simulink model "FTC"  (R2025a)
settings: Solver=ode45  StartTime=0.0  StopTime=10  RelTol=1e-3  EnableMultiTasking=on
values from neighbouring files (symbols this model uses):
  A = [-0.64 1.51 -22.95 9.78 0 ... (first row only)    [thesis_final.m]
  B = [-1.25 3.19 ... (first row only)    [thesis_final.m]
  C = [0.04 0 0 0 0 ... (first row only)    [thesis_final.m]
  E = amp*ones(5,2)    [thesis_final.m]
  fault_type = input('1=abrupt fault ,2= incipient fault,3=intermittent fault:')    [thesis_final.m]
  L = (w*inv(l))'    [thesis_final.m]
  t_fault = input('simulation start time=0s, end time=10s:')    [thesis_final.m]
  W = W'    [thesis_final.m]
undefined symbols (not defined in the file or in its folder): Continuous, K, Kab, Kinc, Kint, Time
libraries: dspsrcs4 x14, simulink x5, ctrlSharedLib x4
settings Model: SimulationMode=accelerator  Creator=Qandeel Fazal  LastModifiedBy=VICTUS
settings SolverCC: MaxConsecutiveZCs=100000  ZeroCrossControl=DisableAll  ZeroCrossAlgorithm=Adaptive  AlgebraicLoopSolver=TrustRegion
settings DataIOCC: LimitDataPoints=on  SaveFormat=Array  ReturnWorkspaceOutputs=off
settings OptimizationCC: EfficientMapNaN2IntZero=off  LifeSpan=inf  SimCompilerOptimization=on
settings DebuggingCC: UnconnectedInputMsg=warning  UnconnectedOutputMsg=warning  UnconnectedLineMsg=warning  SFUnexpectedBacktrackingDiag=warning  SFNoUnconditionalDefaultTransitionDiag=warning  SFExecutionAtInitializationDiag=none  ArithmeticOperatorsInVariantConditions=warning
settings HardwareCC: ProdBitPerPointer=32.0  ProdBitPerSizeT=32.0  ProdBitPerPtrDiffT=32.0  ProdLargestAtomicFloat=None  ProdIntDivRoundTo=Undefined  ProdEndianess=Unspecified  ProdWordSize=32.0  ProdHWDeviceType=32-bit Generic  TargetBitPerPointer=64.0  TargetBitPerSizeT=64.0  TargetBitPerPtrDiffT=64.0  TargetLongLongMode=on  TargetIntDivRoundTo=Zero  TargetEndianess=LittleEndian  TargetWordSize=64.0  TargetHWDeviceType=MATLAB Host  ProdEqTarget=off
settings ModelReferenceCC: EnableRefExpFcnMdlSchedulingChecks=on  PropagateSignalLabelsOutOfModel=off
settings SFSimCC: SimUseLocalCustomCode=off  CustomCodeUndefinedFunction=UseInterfaceOnly
settings RTWCC: RTWUseLocalCustomCode=off  GPUComputeCapability=3.5
settings CodeAppCC: MaxIdLength=128.0  StateflowObjectComments=on
settings GRTTargetCC: TargetLangStandard=C89/C90 (ANSI)  CombineOutputUpdateFcns=off  GRTInterface=on
settings ConfigComp: CovMetricSettings=dw  CovSaveCumulativeToWorkspaceVar=on  CovSaveSingleToWorkspaceVar=on  CovExternalEMLEnable=off  CovSFcnEnable=off

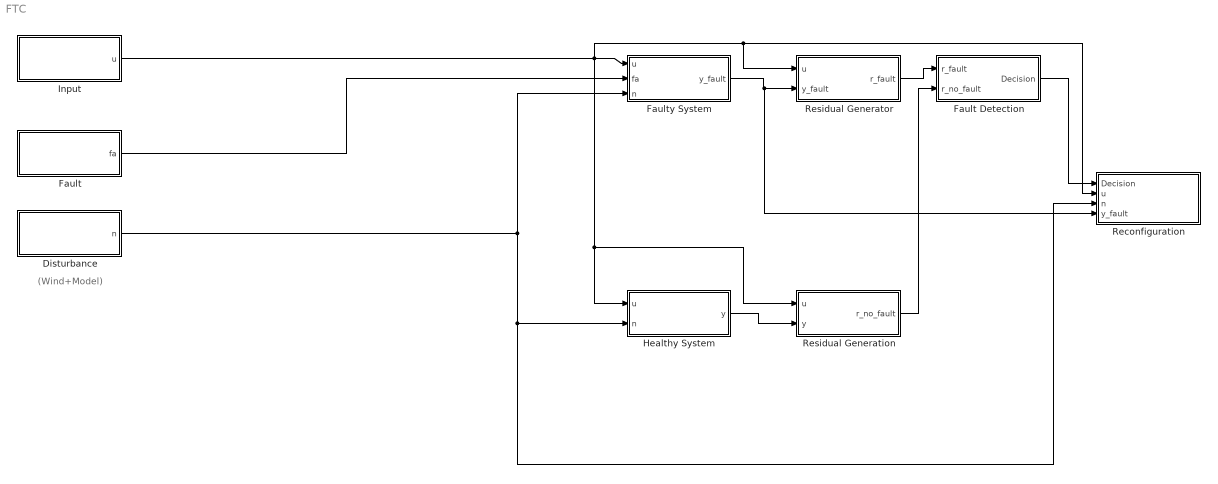
== system FTC ==
  note: (Wind+Model)
  Disturbance : Subsystem
  Fault : Subsystem
  Fault Detection : Subsystem
  Faulty System : Subsystem
  Healthy System : Subsystem
  Input : Subsystem
  Reconfiguration : Subsystem
  Residual Generation : Subsystem
  Residual Generator : Subsystem
  wires:
  Faulty System/1(y_fault) -> Reconfiguration/4(y_fault), Residual Generator/2(y_fault)
  Healthy System/1(y) -> Residual Generation/2(y)
  Fault/1(fa) -> Faulty System/2(fa)
  Residual Generator/1(r_fault) -> Fault Detection/1(r_fault)
  Residual Generation/1(r_no_fault) -> Fault Detection/2(r_no_fault)
  Fault Detection/1(Decision) -> Reconfiguration/1(Decision)
  Input/1(u) -> Reconfiguration/2(u), Residual Generator/1(u), Healthy System/1(u), Residual Generation/1(u), Faulty System/1(u)
  Disturbance/1(n) -> Healthy System/2(n), Reconfiguration/3(n), Faulty System/3(n)

== system FTC/Disturbance ==
  Mux : Mux  Inputs=2
  Scope2 : Scope  Commented=on
      settings: DataLoggingVariableName=ScopeData3  DataLoggingSaveFormat=Array
  To Workspace6 : ToWorkspace  VariableName=n  SaveFormat=Timeseries  SampleTime=-1
      settings: Save2DSignal=2-D array (concatenate along first dimension)
  n(1) : dspsrcs4/Random Source  SrcType=Gaussian  NormMethod=Ziggurat  CltLength=12  MinVal=0  MaxVal=1  MeanVal=0  VarVal=0.1  RepMode=Not repeatable  rawSeed=1  IsInherit=off  SampMode=Continuous  SampTime=1  SampFrame=1  DataType=Double  OutComplex=Real  OutputFrames=on
  n(2) : dspsrcs4/Random Source  SrcType=Gaussian  NormMethod=Ziggurat  CltLength=12  MinVal=0  MaxVal=1  MeanVal=0  VarVal=0.1  RepMode=Not repeatable  rawSeed=1  IsInherit=off  SampMode=Continuous  SampTime=1  SampFrame=1  DataType=Double  OutComplex=Real  OutputFrames=on
  n : Outport
  wires:
  Mux/1 -> n/1, To Workspace6/1, Scope2/1
  n(1)/1 -> Mux/1
  n(2)/1 -> Mux/2

== system FTC/Fault ==
  Constant : Constant  Value=fault_type
  Constant1 : Constant  Value=0
  Constant2 : Constant  Value=0
  Incipient Fault : simulink/Sources/Ramp  slope=1  start=t_fault  X0=0
  Intermittent Fault : DiscretePulseGenerator  PulseType=Time based  Period=3  PulseWidth=4  PhaseDelay=t_fault
  Multiport Switch : MultiPortSwitch  DataPortOrder=Specify indices  SaturateOnIntegerOverflow=off  InputSameDT=off
  Mux : Mux  Inputs=2
  Mux1 : Mux  Inputs=2
  Mux2 : Mux  Inputs=2
  Scope2 : Scope  Commented=on
      settings: DataLoggingVariableName=ScopeData3  DataLoggingSaveFormat=Array
  To Workspace6 : ToWorkspace  VariableName=fa  SaveFormat=Timeseries  SampleTime=-1
      settings: Save2DSignal=2-D array (concatenate along first dimension)
  fa(1) : Step  Time=t_fault  After=0.3  SampleTime=0  VectorParams1D=off
  fa(2) : Step  Time=t_fault  After=0.3  SampleTime=0
  fa : Outport
  wires:
  Mux/1 -> Multiport Switch/2
  fa(1)/1 -> Mux/1
  fa(2)/1 -> Mux/2
  Incipient Fault/1 -> Mux1/1
  Constant1/1 -> Mux1/2
  Multiport Switch/1 -> fa/1, Scope2/1, To Workspace6/1
  Intermittent Fault/1 -> Mux2/1
  Constant2/1 -> Mux2/2
  Mux2/1 -> Multiport Switch/4
  Mux1/1 -> Multiport Switch/3
  Constant/1 -> Multiport Switch/1

== system FTC/Fault Detection ==
  r_fault : Inport
  r_no_fault : Inport  Port=2
  MATLAB Function : MATLAB Function  TreatAsAtomicUnit=on
  Scope8 : Scope  Commented=on  NumInputPorts=4
      settings: TimeSpan=50  ActiveDisplayYMinimum=0  ActiveDisplayYMaximum=1  DataLoggingVariableName=ScopeData11  DataLoggingSaveFormat=Array
  To Workspace1 : ToWorkspace  VariableName=d3  SaveFormat=Timeseries  SampleTime=-1
      settings: Save2DSignal=2-D array (concatenate along first dimension)
  To Workspace2 : ToWorkspace  VariableName=d4  SaveFormat=Timeseries  SampleTime=-1
      settings: Save2DSignal=2-D array (concatenate along first dimension)
  To Workspace3 : ToWorkspace  VariableName=decision  SaveFormat=Timeseries  SampleTime=-1
      settings: Save2DSignal=2-D array (concatenate along first dimension)
  To Workspace5 : ToWorkspace  VariableName=d1  SaveFormat=Timeseries  SampleTime=-1
      settings: Save2DSignal=2-D array (concatenate along first dimension)
  To Workspace8 : ToWorkspace  VariableName=d2  SaveFormat=Timeseries  SampleTime=-1
      settings: Save2DSignal=2-D array (concatenate along first dimension)
  Decision : Outport
  wires:
  MATLAB Function/1(d1) -> Decision/1, To Workspace3/1, Scope8/1, To Workspace5/1
  MATLAB Function/2(d2) -> To Workspace8/1, Scope8/2
  MATLAB Function/3(d3) -> Scope8/3, To Workspace1/1
  MATLAB Function/4(d4) -> Scope8/4, To Workspace2/1
  r_fault/1 -> MATLAB Function/1(r_fault)
  r_no_fault/1 -> MATLAB Function/2(r_no_fault)

== system FTC/Faulty System ==
  u : Inport
  fa : Inport  Port=2
  n : Inport  Port=3
  Mux : Mux  Inputs=2
  Scope2 : Scope  Commented=on
      settings: DataLoggingSaveFormat=Array
  State-Space : StateSpace  A=A  B=[B E]  C=C  D=zeros(5,4)  InitialCondition=[0 ;0;0;0;0]
  Sum5 : Sum  Inputs=|++
  To Workspace6 : ToWorkspace  VariableName=y_fault  SaveFormat=Timeseries  SampleTime=-1
      settings: Save2DSignal=2-D array (concatenate along first dimension)
  y_fault : Outport
  wires:
  fa/1 -> Sum5/2
  Mux/1 -> State-Space/1
  u/1 -> Sum5/1
  Sum5/1 -> Mux/1
  State-Space/1 -> To Workspace6/1, Scope2/1, y_fault/1
  n/1 -> Mux/2

== system FTC/Healthy System ==
  u : Inport
  n : Inport  Port=2
  Mux1 : Mux  Inputs=2
  Scope4 : Scope  Commented=on
      settings: DataLoggingVariableName=ScopeData10  DataLoggingSaveFormat=Array
  State-Space1 : StateSpace  A=A  B=[B E]  C=C  D=zeros(5,4)  InitialCondition=[0 ;0;0;0;0]
  To Workspace4 : ToWorkspace  VariableName=y  SaveFormat=Timeseries  SampleTime=-1
      settings: Save2DSignal=2-D array (concatenate along first dimension)
  y : Outport
  wires:
  u/1 -> Mux1/1
  Mux1/1 -> State-Space1/1
  n/1 -> Mux1/2
  State-Space1/1 -> y/1, To Workspace4/1, Scope4/1

== system FTC/Input ==
  Scope2 : Scope  Commented=on
      settings: DataLoggingVariableName=ScopeData3  DataLoggingSaveFormat=Array
  To Workspace6 : ToWorkspace  VariableName=u  SaveFormat=Timeseries  SampleTime=-1
      settings: Save2DSignal=2-D array (concatenate along first dimension)
  u(1)1 : Step  Before=[0 0]  After=[5 5]  SampleTime=0
  u : Outport
  wires:
  u(1)1/1 -> Scope2/1, u/1, To Workspace6/1

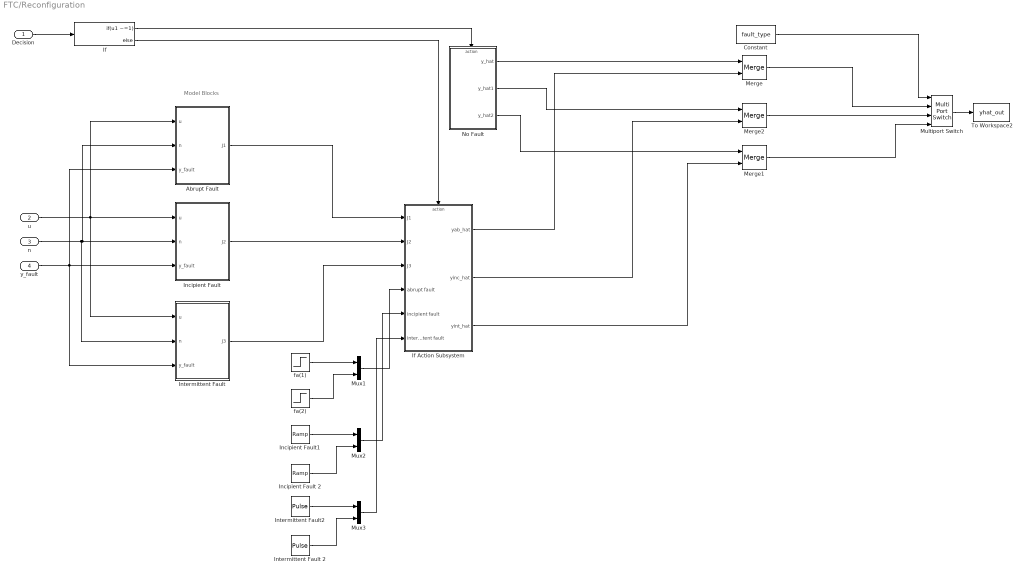
== system FTC/Reconfiguration ==
  note: Model Blocks
  Decision : Inport
  u : Inport  Port=2
  n : Inport  Port=3
  y_fault : Inport  Port=4
  Abrupt Fault : Subsystem
  Constant : Constant  Value=fault_type
  If : If  IfExpression=u1 ~=1
  If Action Subsystem : Subsystem  TreatAsAtomicUnit=on
  Incipient Fault : Subsystem
  Incipient Fault 2 : simulink/Sources/Ramp  slope=0  start=t_fault  InitialOutput=0
  Incipient Fault1 : simulink/Sources/Ramp  slope=1  start=5  InitialOutput=0
  Intermittent Fault : Subsystem
  Intermittent Fault 2 : DiscretePulseGenerator  PulseType=Time based  Amplitude=0  Period=10  PulseWidth=5
  Intermittent Fault2 : DiscretePulseGenerator  PulseType=Time based  PulseWidth=1.5  PhaseDelay=5
  Merge : Merge
  Merge1 : Merge
  Merge2 : Merge
  Multiport Switch : MultiPortSwitch  DataPortOrder=Specify indices  SaturateOnIntegerOverflow=off  InputSameDT=off
  Mux1 : Mux  Inputs=2
  Mux2 : Mux  Inputs=2
  Mux3 : Mux  Inputs=2
  No Fault : Subsystem  TreatAsAtomicUnit=on
  To Workspace2 : ToWorkspace  VariableName=yhat_out  SaveFormat=Timeseries  SampleTime=-1
  fa(1) : Step  Time=5  After=0.3  SampleTime=0  VectorParams1D=off
  fa(2) : Step  Time=t_fault  After=0  SampleTime=0
  wires:
  Decision/1 -> If/1
  If/2 -> If Action Subsystem/Action
  If/1 -> No Fault/Action
  Intermittent Fault/1(J3) -> If Action Subsystem/3(J3)
  u/1 -> Intermittent Fault/1(u), Abrupt Fault/1(u), Incipient Fault/1(u)
  n/1 -> Intermittent Fault/2(n), Abrupt Fault/2(n), Incipient Fault/2(n)
  y_fault/1 -> Intermittent Fault/3(y_fault), Abrupt Fault/3(y_fault), Incipient Fault/3(y_fault)
  Incipient Fault/1(J2) -> If Action Subsystem/2(J2)
  Abrupt Fault/1(J1) -> If Action Subsystem/1(J1)
  If Action Subsystem/1(yab_hat) -> Merge/2
  No Fault/1(y_hat) -> Merge/1
  If Action Subsystem/2(yinc_hat) -> Merge2/2
  No Fault/2(y_hat1) -> Merge2/1
  If Action Subsystem/3(yint_hat) -> Merge1/2
  No Fault/3(y_hat2) -> Merge1/1
  Constant/1 -> Multiport Switch/1
  Merge/1 -> Multiport Switch/2
  Merge2/1 -> Multiport Switch/3
  Merge1/1 -> Multiport Switch/4
  Multiport Switch/1 -> To Workspace2/1
  Mux1/1 -> If Action Subsystem/4(abrupt fault)
  fa(1)/1 -> Mux1/1
  fa(2)/1 -> Mux1/2
  Incipient Fault1/1 -> Mux2/1
  Incipient Fault 2/1 -> Mux2/2
  Intermittent Fault2/1 -> Mux3/1
  Intermittent Fault 2/1 -> Mux3/2
  Mux3/1 -> If Action Subsystem/6(intermittent fault)
  Mux2/1 -> If Action Subsystem/5(incipient fault)

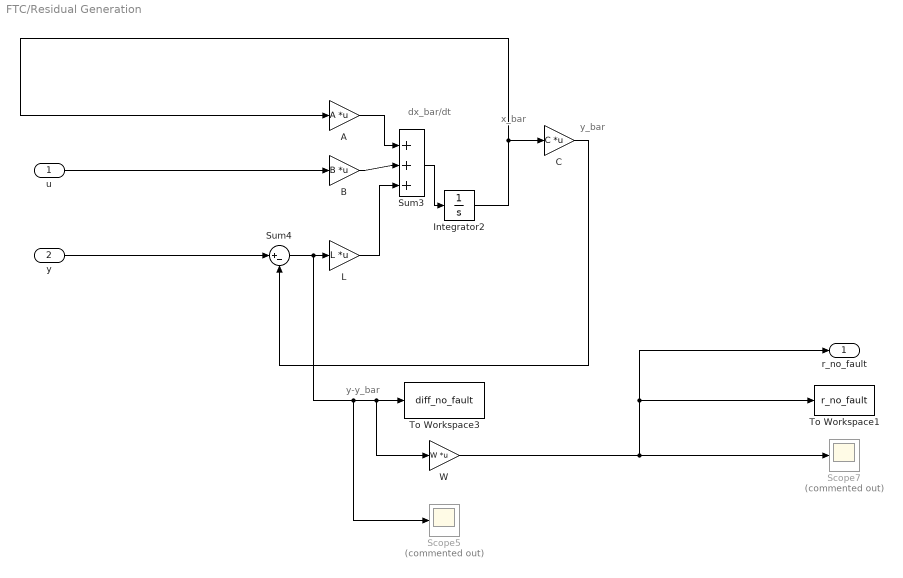
== system FTC/Residual Generation ==
  note: y-y_bar
  note: y_bar
  note: x_bar
  note: dx_bar/dt
  u : Inport
  y : Inport  Port=2
  "A " : Gain  Gain=A  Multiplication=Matrix(K*u)
  B : Gain  Gain=B  Multiplication=Matrix(K*u)
  C : Gain  Gain=C  Multiplication=Matrix(K*u)
  Integrator2 : Integrator
  "L " : Gain  Gain=L  Multiplication=Matrix(K*u)
  Scope5 : Scope  Commented=on
      settings: TimeSpan=50  ActiveDisplayYMinimum=-0.4  ActiveDisplayYMaximum=0.4  DataLoggingVariableName=ScopeData12  DataLoggingSaveFormat=Array
  Scope7 : Scope  Commented=on
      settings: TimeSpan=50  ActiveDisplayYMinimum=-0.4  ActiveDisplayYMaximum=0.80000000000000016  DataLoggingVariableName=ScopeData13  DataLoggingSaveFormat=Array
  Sum3 : Sum  Inputs=|+++
  Sum4 : Sum  Inputs=|+-
  To Workspace1 : ToWorkspace  VariableName=r_no_fault  SaveFormat=Timeseries  SampleTime=-1
      settings: Save2DSignal=2-D array (concatenate along first dimension)
  To Workspace3 : ToWorkspace  VariableName=diff_no_fault  SaveFormat=Timeseries  SampleTime=-1
      settings: Save2DSignal=2-D array (concatenate along first dimension)
  W : Gain  Gain=W  Multiplication=Matrix(K*u)
  r_no_fault : Outport
  wires:
  u/1 -> B/1
  B/1 -> Sum3/2
  "A "/1 -> Sum3/1
  C/1 -> Sum4/2
  Sum3/1 -> Integrator2/1
  "L "/1 -> Sum3/3
  Integrator2/1 -> C/1, "A "/1
  y/1 -> Sum4/1
  Sum4/1 -> Scope5/1, W/1, To Workspace3/1, "L "/1
  W/1 -> Scope7/1, r_no_fault/1, To Workspace1/1

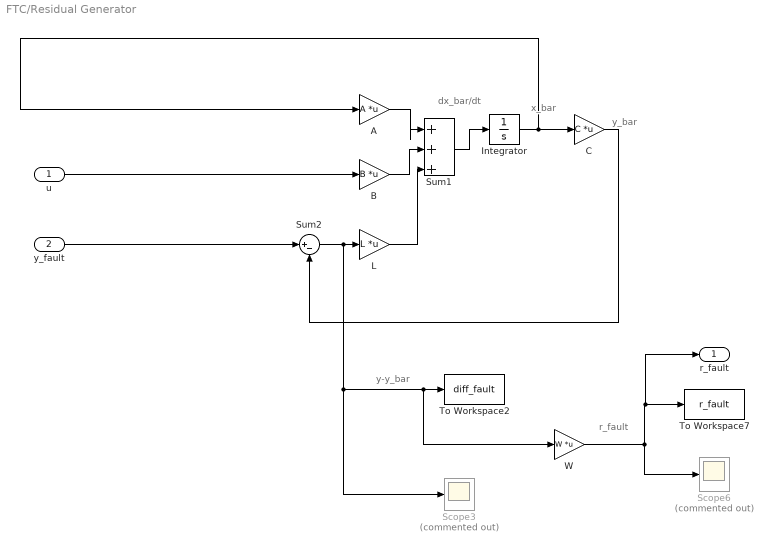
== system FTC/Residual Generator ==
  note: y_bar
  note: y-y_bar
  note: x_bar
  note: dx_bar/dt
  note: r_fault
  u : Inport
  y_fault : Inport  Port=2
  A : Gain  Gain=A  Multiplication=Matrix(K*u)
  B : Gain  Gain=B  Multiplication=Matrix(K*u)
  C : Gain  Gain=C  Multiplication=Matrix(K*u)
  Integrator : Integrator
  L : Gain  Gain=L  Multiplication=Matrix(K*u)
  Scope3 : Scope  Commented=on
      settings: TimeSpan=50  ActiveDisplayYMinimum=-0.4  ActiveDisplayYMaximum=0.80000000000000016  DataLoggingSaveFormat=Array
  Scope6 : Scope  Commented=on
      settings: TimeSpan=50  ActiveDisplayYMinimum=-100  ActiveDisplayYMaximum=600  DataLoggingVariableName=ScopeData9  DataLoggingSaveFormat=Array
  Sum1 : Sum  Inputs=|+++
  Sum2 : Sum  Inputs=|+-
  To Workspace2 : ToWorkspace  VariableName=diff_fault  SaveFormat=Timeseries  SampleTime=-1
      settings: Save2DSignal=2-D array (concatenate along first dimension)
  To Workspace7 : ToWorkspace  VariableName=r_fault  SaveFormat=Timeseries  SampleTime=-1
      settings: Save2DSignal=2-D array (concatenate along first dimension)
  W : Gain  Gain=W  Multiplication=Matrix(K*u)
  r_fault : Outport
  wires:
  B/1 -> Sum1/2
  A/1 -> Sum1/1
  C/1 -> Sum2/2
  Sum1/1 -> Integrator/1
  L/1 -> Sum1/3
  Integrator/1 -> C/1, A/1
  Sum2/1 -> W/1, To Workspace2/1, Scope3/1, L/1
  y_fault/1 -> Sum2/1
  u/1 -> B/1
  W/1 -> Scope6/1, r_fault/1, To Workspace7/1

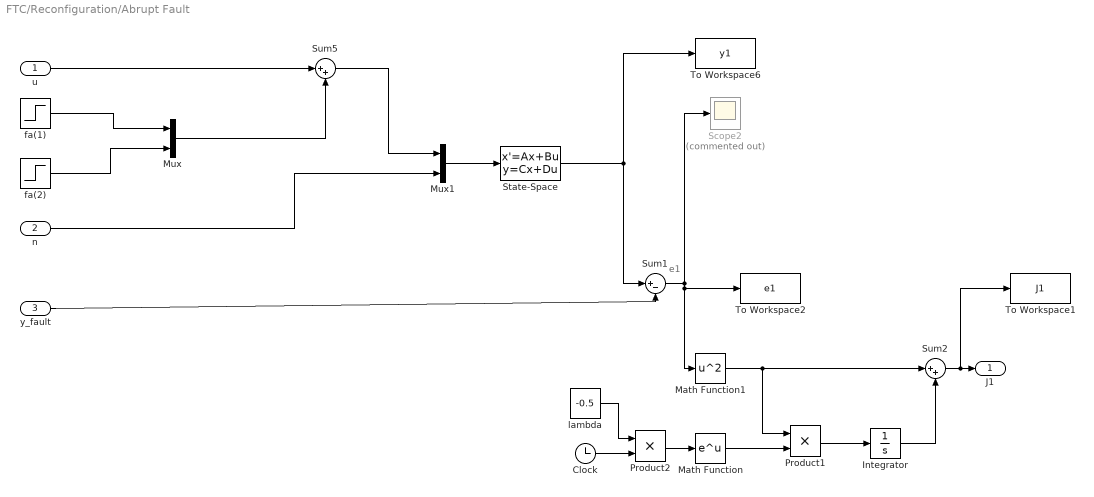
== system FTC/Reconfiguration/Abrupt Fault ==
  note: e1
  u : Inport
  n : Inport  Port=2
  y_fault : Inport  Port=3
  Clock : Clock
  Integrator : Integrator
  Math Function : Math  SignedPower=on
  Math Function1 : Math  Operator=square  SignedPower=on
  Mux : Mux  Inputs=2
  Mux1 : Mux  Inputs=2
  Product1 : Product
  Product2 : Product
  Scope2 : Scope  Commented=on
      settings: DataLoggingVariableName=ScopeData2  DataLoggingSaveFormat=Array
  State-Space : StateSpace  A=A  B=[B E]  C=C  D=zeros(5,4)  InitialCondition=[0 ;0;0;0;0]
  Sum1 : Sum  Inputs=|+-
  Sum2 : Sum  Inputs=|++
  Sum5 : Sum  Inputs=|++
  To Workspace1 : ToWorkspace  VariableName=J1  SaveFormat=Timeseries  SampleTime=-1
      settings: Save2DSignal=2-D array (concatenate along first dimension)
  To Workspace2 : ToWorkspace  VariableName=e1  SaveFormat=Timeseries  SampleTime=-1
      settings: Save2DSignal=2-D array (concatenate along first dimension)
  To Workspace6 : ToWorkspace  VariableName=y1  SaveFormat=Timeseries  SampleTime=-1
      settings: Save2DSignal=2-D array (concatenate along first dimension)
  fa(1) : Step  Time=5  After=0.3  SampleTime=0  VectorParams1D=off
  fa(2) : Step  Time=t_fault  After=0  SampleTime=0
  lambda : Constant  Value=-0.5
  J1 : Outport
  wires:
  n/1 -> Mux1/2
  u/1 -> Sum5/1
  Sum5/1 -> Mux1/1
  Mux1/1 -> State-Space/1
  State-Space/1 -> To Workspace6/1, Sum1/1
  Mux/1 -> Sum5/2
  fa(1)/1 -> Mux/1
  y_fault/1 -> Sum1/2
  Sum1/1 -> Math Function1/1, To Workspace2/1, Scope2/1
  fa(2)/1 -> Mux/2
  Math Function1/1 -> Sum2/1, Product1/1
  Clock/1 -> Product2/2
  lambda/1 -> Product2/1
  Product2/1 -> Math Function/1
  Math Function/1 -> Product1/2
  Product1/1 -> Integrator/1
  Integrator/1 -> Sum2/2
  Sum2/1 -> To Workspace1/1, J1/1

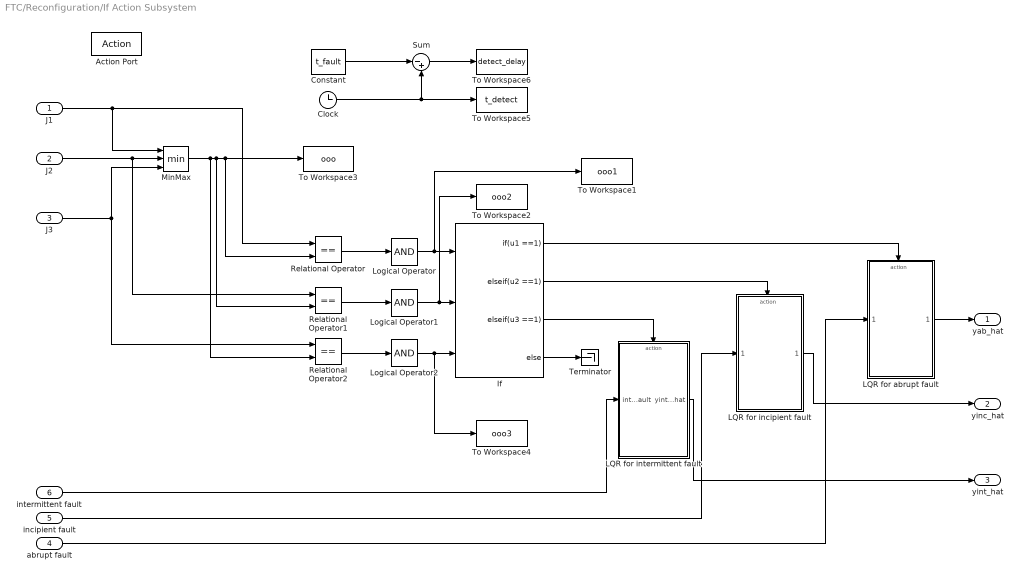
== system FTC/Reconfiguration/If Action Subsystem ==
  J1 : Inport
  J2 : Inport  Port=2
  J3 : Inport  Port=3
  abrupt fault : Inport  Port=4
  incipient fault : Inport  Port=5
  intermittent fault : Inport  Port=6
  Action Port : ActionPort  ActionPortLabel=else { }
  Clock : Clock
  Constant : Constant  Value=t_fault
  If : If  NumInputs=3  IfExpression=u1 ==1  ElseIfExpressions=u2 ==1,u3 ==1
  LQR for abrupt fault : Subsystem  TreatAsAtomicUnit=on
  LQR for incipient fault : Subsystem  TreatAsAtomicUnit=on
  LQR for intermittent fault : Subsystem  TreatAsAtomicUnit=on
  Logical Operator : Logic  Inputs=1  AllPortsSameDT=off  OutDataTypeStr=boolean
  Logical Operator1 : Logic  Inputs=1  AllPortsSameDT=off  OutDataTypeStr=boolean
  Logical Operator2 : Logic  Inputs=1  AllPortsSameDT=off  OutDataTypeStr=boolean
  MinMax : MinMax  Inputs=3
  Relational Operator : RelationalOperator  Operator===  OutDataTypeStr=boolean  InputSameDT=off
  Relational Operator1 : RelationalOperator  Operator===  OutDataTypeStr=boolean  InputSameDT=off
  Relational Operator2 : RelationalOperator  Operator===  OutDataTypeStr=boolean  InputSameDT=off
  Sum : Sum  Inputs=|-+
  Terminator : Terminator
  To Workspace1 : ToWorkspace  VariableName=ooo1  SaveFormat=Timeseries  SampleTime=-1
      settings: Save2DSignal=2-D array (concatenate along first dimension)
  To Workspace2 : ToWorkspace  VariableName=ooo2  SaveFormat=Timeseries  SampleTime=-1
      settings: Save2DSignal=2-D array (concatenate along first dimension)
  To Workspace3 : ToWorkspace  VariableName=ooo  SaveFormat=Timeseries  SampleTime=-1
      settings: Save2DSignal=2-D array (concatenate along first dimension)
  To Workspace4 : ToWorkspace  VariableName=ooo3  SaveFormat=Timeseries  SampleTime=-1
      settings: Save2DSignal=2-D array (concatenate along first dimension)
  To Workspace5 : ToWorkspace  VariableName=t_detect  SaveFormat=Timeseries  SampleTime=-1
      settings: Save2DSignal=2-D array (concatenate along first dimension)
  To Workspace6 : ToWorkspace  VariableName=detect_delay  SaveFormat=Timeseries  SampleTime=-1
      settings: Save2DSignal=2-D array (concatenate along first dimension)
  yab_hat : Outport
  yinc_hat : Outport  Port=2
  yint_hat : Outport  Port=3
  wires:
  J1/1 -> MinMax/1, Relational Operator/1
  J2/1 -> Relational Operator1/1, MinMax/2
  J3/1 -> MinMax/3, Relational Operator2/1
  MinMax/1 -> Relational Operator2/2, Relational Operator1/2, Relational Operator/2, To Workspace3/1
  If/1 -> LQR for abrupt fault/Action
  If/2 -> LQR for incipient fault/Action
  If/3 -> LQR for intermittent fault/Action
  If/4 -> Terminator/1
  Relational Operator/1 -> Logical Operator/1
  Logical Operator/1 -> To Workspace1/1, If/1
  Relational Operator1/1 -> Logical Operator1/1
  Logical Operator1/1 -> To Workspace2/1, If/2
  Logical Operator2/1 -> To Workspace4/1, If/3
  Relational Operator2/1 -> Logical Operator2/1
  Clock/1 -> Sum/2, To Workspace5/1
  Constant/1 -> Sum/1
  Sum/1 -> To Workspace6/1
  abrupt fault/1 -> LQR for abrupt fault/1(abrupt fault)
  incipient fault/1 -> LQR for incipient fault/1(incipient fault)
  intermittent fault/1 -> LQR for intermittent fault/1(intermittent fault)
  LQR for abrupt fault/1(yab_hat) -> yab_hat/1
  LQR for incipient fault/1(yinc_hat) -> yinc_hat/1
  LQR for intermittent fault/1(yint_hat) -> yint_hat/1

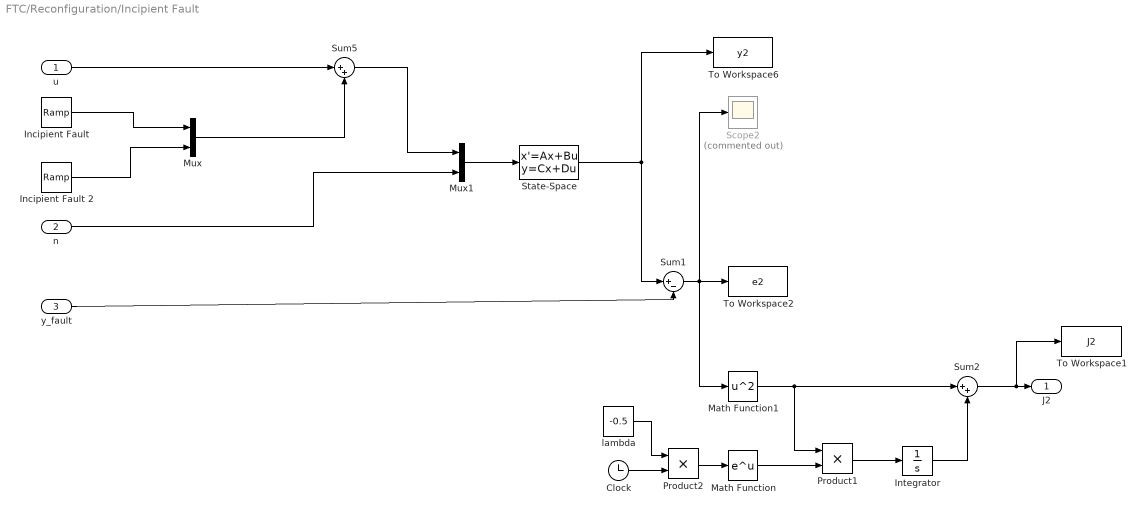
== system FTC/Reconfiguration/Incipient Fault ==
  u : Inport
  n : Inport  Port=2
  y_fault : Inport  Port=3
  Clock : Clock
  Incipient Fault : simulink/Sources/Ramp  slope=1  start=5  X0=0
  Incipient Fault 2 : simulink/Sources/Ramp  slope=0  start=t_fault  X0=0
  Integrator : Integrator
  Math Function : Math  SignedPower=on
  Math Function1 : Math  Operator=square  SignedPower=on
  Mux : Mux  Inputs=2
  Mux1 : Mux  Inputs=2
  Product1 : Product
  Product2 : Product
  Scope2 : Scope  Commented=on
      settings: DataLoggingVariableName=ScopeData2  DataLoggingSaveFormat=Array
  State-Space : StateSpace  A=A  B=[B E]  C=C  D=zeros(5,4)  InitialCondition=[0 ;0;0;0;0]
  Sum1 : Sum  Inputs=|+-
  Sum2 : Sum  Inputs=|++
  Sum5 : Sum  Inputs=|++
  To Workspace1 : ToWorkspace  VariableName=J2  SaveFormat=Timeseries  SampleTime=-1
      settings: Save2DSignal=2-D array (concatenate along first dimension)
  To Workspace2 : ToWorkspace  VariableName=e2  SaveFormat=Timeseries  SampleTime=-1
      settings: Save2DSignal=2-D array (concatenate along first dimension)
  To Workspace6 : ToWorkspace  VariableName=y2  SaveFormat=Timeseries  SampleTime=-1
      settings: Save2DSignal=2-D array (concatenate along first dimension)
  lambda : Constant  Value=-0.5
  J2 : Outport
  wires:
  n/1 -> Mux1/2
  u/1 -> Sum5/1
  Sum5/1 -> Mux1/1
  Mux1/1 -> State-Space/1
  State-Space/1 -> To Workspace6/1, Sum1/1
  Mux/1 -> Sum5/2
  Incipient Fault/1 -> Mux/1
  Incipient Fault 2/1 -> Mux/2
  y_fault/1 -> Sum1/2
  Sum1/1 -> To Workspace2/1, Math Function1/1, Scope2/1
  Math Function1/1 -> Sum2/1, Product1/1
  Clock/1 -> Product2/2
  lambda/1 -> Product2/1
  Product2/1 -> Math Function/1
  Math Function/1 -> Product1/2
  Product1/1 -> Integrator/1
  Integrator/1 -> Sum2/2
  Sum2/1 -> To Workspace1/1, J2/1

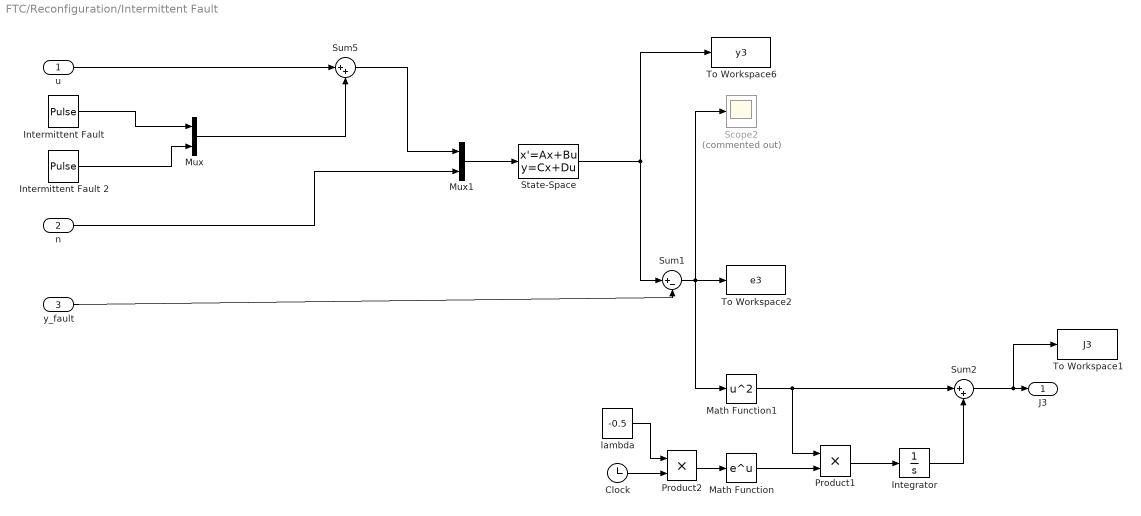
== system FTC/Reconfiguration/Intermittent Fault ==
  u : Inport
  n : Inport  Port=2
  y_fault : Inport  Port=3
  Clock : Clock
  Integrator : Integrator
  Intermittent Fault : DiscretePulseGenerator  PulseType=Time based  PulseWidth=1.5  PhaseDelay=5
  Intermittent Fault 2 : DiscretePulseGenerator  PulseType=Time based  Amplitude=0  Period=10  PulseWidth=5
  Math Function : Math  SignedPower=on
  Math Function1 : Math  Operator=square  SignedPower=on
  Mux : Mux  Inputs=2
  Mux1 : Mux  Inputs=2
  Product1 : Product
  Product2 : Product
  Scope2 : Scope  Commented=on
      settings: DataLoggingVariableName=ScopeData2  DataLoggingSaveFormat=Array
  State-Space : StateSpace  A=A  B=[B E]  C=C  D=zeros(5,4)  InitialCondition=[0 ;0;0;0;0]
  Sum1 : Sum  Inputs=|+-
  Sum2 : Sum  Inputs=|++
  Sum5 : Sum  Inputs=|++
  To Workspace1 : ToWorkspace  VariableName=J3  SaveFormat=Timeseries  SampleTime=-1
      settings: Save2DSignal=2-D array (concatenate along first dimension)
  To Workspace2 : ToWorkspace  VariableName=e3  SaveFormat=Timeseries  SampleTime=-1
      settings: Save2DSignal=2-D array (concatenate along first dimension)
  To Workspace6 : ToWorkspace  VariableName=y3  SaveFormat=Timeseries  SampleTime=-1
      settings: Save2DSignal=2-D array (concatenate along first dimension)
  lambda : Constant  Value=-0.5
  J3 : Outport
  wires:
  n/1 -> Mux1/2
  u/1 -> Sum5/1
  Sum5/1 -> Mux1/1
  Mux1/1 -> State-Space/1
  State-Space/1 -> To Workspace6/1, Sum1/1
  Mux/1 -> Sum5/2
  Intermittent Fault/1 -> Mux/1
  Intermittent Fault 2/1 -> Mux/2
  y_fault/1 -> Sum1/2
  Sum1/1 -> To Workspace2/1, Math Function1/1, Scope2/1
  Math Function1/1 -> Sum2/1, Product1/1
  Clock/1 -> Product2/2
  lambda/1 -> Product2/1
  Product2/1 -> Math Function/1
  Math Function/1 -> Product1/2
  Product1/1 -> Integrator/1
  Integrator/1 -> Sum2/2
  Sum2/1 -> To Workspace1/1, J3/1

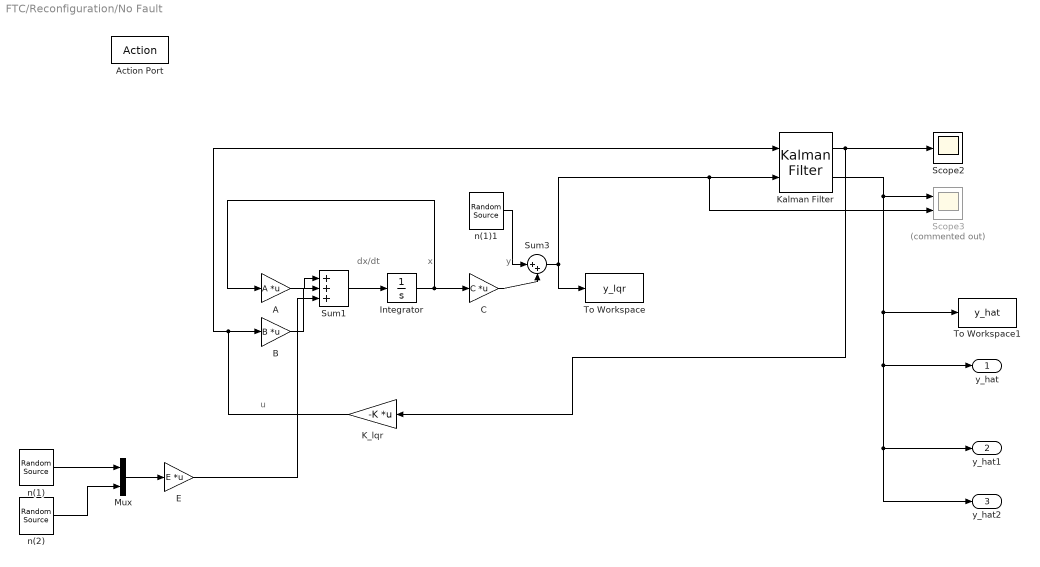
== system FTC/Reconfiguration/No Fault ==
  note: u
  note: y
  note: x
  note: dx/dt
  Action Port : ActionPort  ActionPortLabel=if { }
  A : Gain  Gain=A  Multiplication=Matrix(K*u)
  B : Gain  Gain=B  Multiplication=Matrix(K*u)
  C : Gain  Gain=C  Multiplication=Matrix(K*u)
  E : Gain  Gain=E  Multiplication=Matrix(K*u)
  Integrator : Integrator  InitialCondition=[2;0;0;0;0]
  K_lqr : Gain  Gain=-K  Multiplication=Matrix(K*u)
  Kalman Filter : ctrlSharedLib/Kalman Filter  TimeDomain=Continuous-Time  UseCurrentEstimator=on  ModelSource=Individual A, B, C, D matrices  ModelSourceVariable=ss(0.95,1,1,0,1)  A=A  B=B  C=C  D=zeros(5,2)  NumberOfStates=1  NumberOfInputs=1  NumberOfOutputs=1  InitialEstimateSource=Dialog  X0=[2;0;0;0;0]  P0=10  UseK=off  UseGH=off  NumberOfProcessNoiseInputs=1  G=1  TimeInvariantG=on  H=0  TimeInvariantH=on  Q=0.0001*eye(5)  TimeInvariantQ=on  R=0.0001*eye(5)  TimeInvariantR=on  N=0  TimeInvariantN=on  AddInputPort=on  AddEnablePort=off  ExternalReset=none  OutputEstimatedY=on  OutputP=off  Ts=-1
  Mux : Mux  Inputs=2
  Scope2 : Scope
      settings: TimeSpan=14.81551052143918  ActiveDisplayYMinimum=-0.2  ActiveDisplayYMaximum=0.2  DataLoggingVariableName=ScopeData4  DataLoggingSaveFormat=Array
  Scope3 : Scope  Commented=on  NumInputPorts=2
      settings: TimeSpan=14.81551052143918  ActiveDisplayYMinimum=-4  ActiveDisplayYMaximum=3  DataLoggingVariableName=ScopeData5  DataLoggingSaveFormat=Array
  Sum1 : Sum  Inputs=|+++
  Sum3 : Sum  Inputs=|++
  To Workspace : ToWorkspace  VariableName=y_lqr  SaveFormat=Timeseries  SampleTime=-1
  To Workspace1 : ToWorkspace  VariableName=y_hat  SaveFormat=Timeseries  SampleTime=-1
  n(1) : dspsrcs4/Random Source  SrcType=Gaussian  NormMethod=Ziggurat  CltLength=12  MinVal=0  MaxVal=1  MeanVal=0  VarVal=0.1  RepMode=Not repeatable  rawSeed=1  IsInherit=off  SampMode=Continuous  SampTime=1  SampFrame=1  DataType=Double  OutComplex=Real  OutputFrames=on
  n(1)1 : dspsrcs4/Random Source  SrcType=Gaussian  NormMethod=Ziggurat  CltLength=12  MinVal=0  MaxVal=1  MeanVal=0  VarVal=0.1  RepMode=Not repeatable  rawSeed=1  IsInherit=off  SampMode=Continuous  SampTime=1  SampFrame=1  DataType=Double  OutComplex=Real  OutputFrames=on
  n(2) : dspsrcs4/Random Source  SrcType=Gaussian  NormMethod=Ziggurat  CltLength=12  MinVal=0  MaxVal=1  MeanVal=0  VarVal=0.1  RepMode=Not repeatable  rawSeed=1  IsInherit=off  SampMode=Continuous  SampTime=1  SampFrame=1  DataType=Double  OutComplex=Real  OutputFrames=on
  y_hat : Outport
  y_hat1 : Outport  Port=2
  y_hat2 : Outport  Port=3
  wires:
  B/1 -> Sum1/2
  A/1 -> Sum1/1
  Sum1/1 -> Integrator/1
  Integrator/1 -> C/1, A/1
  n(1)/1 -> Mux/1
  n(2)/1 -> Mux/2
  Mux/1 -> E/1
  K_lqr/1 -> Kalman Filter/1, B/1
  Kalman Filter/1 -> Scope2/1, K_lqr/1
  E/1 -> Sum1/3
  C/1 -> Sum3/2
  n(1)1/1 -> Sum3/1
  Sum3/1 -> To Workspace/1, Scope3/2, Kalman Filter/2
  Kalman Filter/2 -> y_hat1/1, y_hat2/1, y_hat/1, To Workspace1/1, Scope3/1

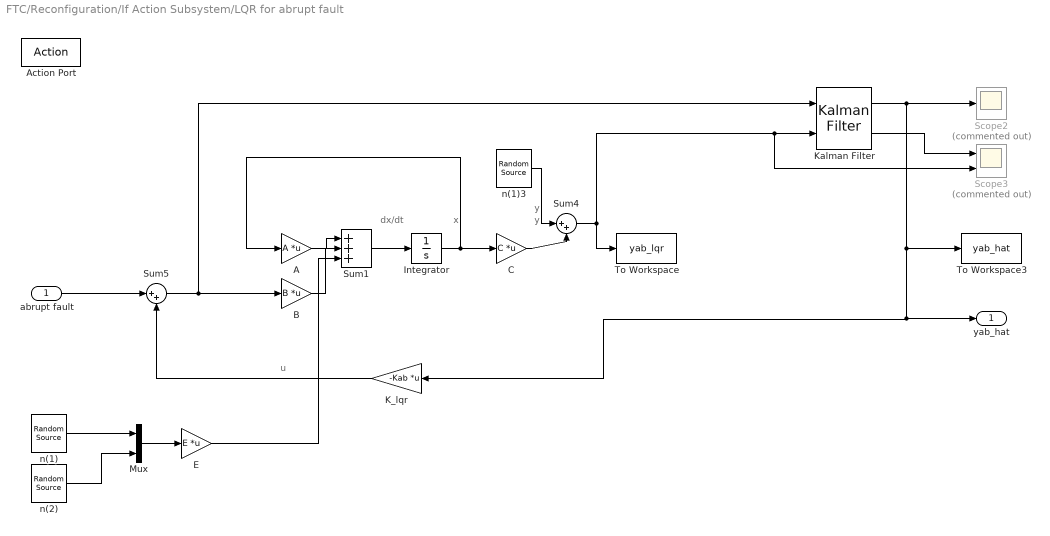
== system FTC/Reconfiguration/If Action Subsystem/LQR for abrupt fault ==
  note: u
  note: y
  note: x
  note: dx/dt
  note: y
  abrupt fault : Inport
  Action Port : ActionPort  ActionPortLabel=if { }
  A : Gain  Gain=A  Multiplication=Matrix(K*u)
  B : Gain  Gain=B  Multiplication=Matrix(K*u)
  C : Gain  Gain=C  Multiplication=Matrix(K*u)
  E : Gain  Gain=E  Multiplication=Matrix(K*u)
  Integrator : Integrator  InitialCondition=[2;0;0;0;0]
  K_lqr : Gain  Gain=-Kab  Multiplication=Matrix(K*u)
  Kalman Filter : ctrlSharedLib/Kalman Filter  TimeDomain=Continuous-Time  UseCurrentEstimator=on  ModelSource=Individual A, B, C, D matrices  ModelSourceVariable=ss(0.95,1,1,0,1)  A=A  B=B  C=C  D=zeros(5,2)  NumberOfStates=1  NumberOfInputs=1  NumberOfOutputs=1  InitialEstimateSource=Dialog  X0=zeros(5,1)  P0=10  UseK=off  UseGH=off  NumberOfProcessNoiseInputs=1  G=1  TimeInvariantG=on  H=0  TimeInvariantH=on  Q=0.001*eye(5)  TimeInvariantQ=on  R=0.001*eye(5)  TimeInvariantR=on  N=0  TimeInvariantN=on  AddInputPort=on  AddEnablePort=off  ExternalReset=none  OutputEstimatedY=on  OutputP=off  Ts=-1
  Mux : Mux  Inputs=2
  Scope2 : Scope  Commented=on
      settings: TimeSpan=14.81551052143918  ActiveDisplayYMinimum=-0.60000000000000009  ActiveDisplayYMaximum=0.60000000000000009  DataLoggingVariableName=ScopeData15  DataLoggingSaveFormat=Array
  Scope3 : Scope  Commented=on  NumInputPorts=2
      settings: TimeSpan=14.81551052143918  ActiveDisplayYMinimum=-4  ActiveDisplayYMaximum=3  DataLoggingVariableName=ScopeData16  DataLoggingSaveFormat=Array
  Sum1 : Sum  Inputs=|+++
  Sum4 : Sum  Inputs=|++
  Sum5 : Sum  Inputs=|++
  To Workspace : ToWorkspace  VariableName=yab_lqr  SaveFormat=Timeseries  SampleTime=-1
  To Workspace3 : ToWorkspace  VariableName=yab_hat  SaveFormat=Timeseries  SampleTime=-1
  n(1) : dspsrcs4/Random Source  SrcType=Gaussian  NormMethod=Ziggurat  CltLength=12  MinVal=0  MaxVal=1  MeanVal=0  VarVal=0.1  RepMode=Not repeatable  rawSeed=1  IsInherit=off  SampMode=Continuous  SampTime=1  SampFrame=1  DataType=Double  OutComplex=Real  OutputFrames=on
  n(1)3 : dspsrcs4/Random Source  SrcType=Gaussian  NormMethod=Ziggurat  CltLength=12  MinVal=0  MaxVal=1  MeanVal=0  VarVal=0.1  RepMode=Not repeatable  rawSeed=1  IsInherit=off  SampMode=Continuous  SampTime=1  SampFrame=1  DataType=Double  OutComplex=Real  OutputFrames=on
  n(2) : dspsrcs4/Random Source  SrcType=Gaussian  NormMethod=Ziggurat  CltLength=12  MinVal=0  MaxVal=1  MeanVal=0  VarVal=0.1  RepMode=Not repeatable  rawSeed=1  IsInherit=off  SampMode=Continuous  SampTime=1  SampFrame=1  DataType=Double  OutComplex=Real  OutputFrames=on
  yab_hat : Outport
  wires:
  B/1 -> Sum1/2
  A/1 -> Sum1/1
  Sum1/1 -> Integrator/1
  Integrator/1 -> C/1, A/1
  n(1)/1 -> Mux/1
  n(2)/1 -> Mux/2
  Mux/1 -> E/1
  Kalman Filter/1 -> To Workspace3/1, yab_hat/1, K_lqr/1, Scope2/1
  Kalman Filter/2 -> Scope3/1
  E/1 -> Sum1/3
  n(1)3/1 -> Sum4/1
  C/1 -> Sum4/2
  Sum4/1 -> Scope3/2, Kalman Filter/2, To Workspace/1
  Sum5/1 -> Kalman Filter/1, B/1
  abrupt fault/1 -> Sum5/1
  K_lqr/1 -> Sum5/2

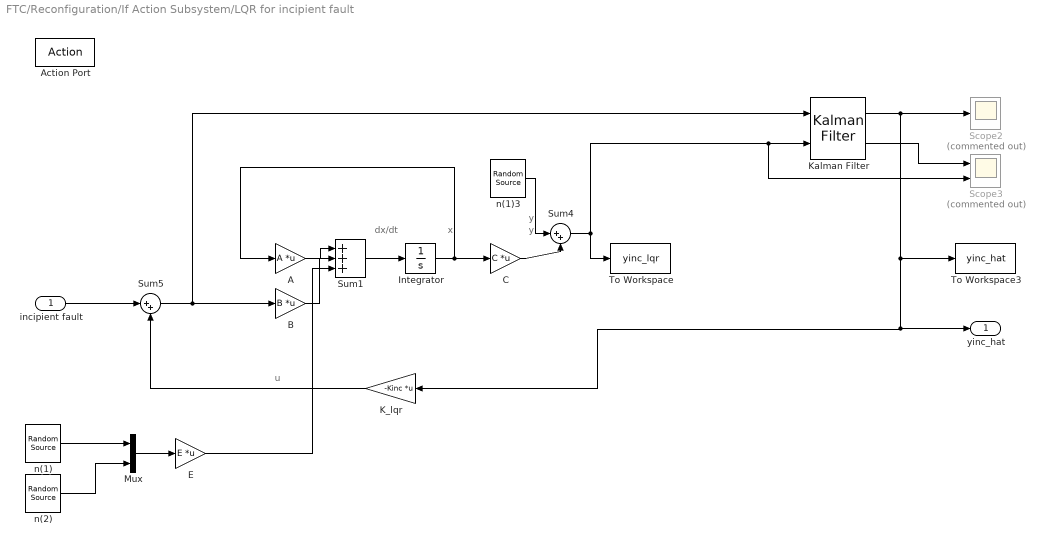
== system FTC/Reconfiguration/If Action Subsystem/LQR for incipient fault ==
  note: u
  note: y
  note: x
  note: dx/dt
  note: y
  incipient fault : Inport
  Action Port : ActionPort  ActionPortLabel=elseif { }
  A : Gain  Gain=A  Multiplication=Matrix(K*u)
  B : Gain  Gain=B  Multiplication=Matrix(K*u)
  C : Gain  Gain=C  Multiplication=Matrix(K*u)
  E : Gain  Gain=E  Multiplication=Matrix(K*u)
  Integrator : Integrator  InitialCondition=[2;0;0;0;0]
  K_lqr : Gain  Gain=-Kinc  Multiplication=Matrix(K*u)
  Kalman Filter : ctrlSharedLib/Kalman Filter  TimeDomain=Continuous-Time  UseCurrentEstimator=on  ModelSource=Individual A, B, C, D matrices  ModelSourceVariable=ss(0.95,1,1,0,1)  A=A  B=B  C=C  D=zeros(5,2)  NumberOfStates=1  NumberOfInputs=1  NumberOfOutputs=1  InitialEstimateSource=Dialog  X0=zeros(5,1)  P0=10  UseK=off  UseGH=off  NumberOfProcessNoiseInputs=1  G=1  TimeInvariantG=on  H=0  TimeInvariantH=on  Q=0.001*eye(5)  TimeInvariantQ=on  R=0.001*eye(5)  TimeInvariantR=on  N=0  TimeInvariantN=on  AddInputPort=on  AddEnablePort=off  ExternalReset=none  OutputEstimatedY=on  OutputP=off  Ts=-1
  Mux : Mux  Inputs=2
  Scope2 : Scope  Commented=on
      settings: TimeSpan=14.81551052143918  ActiveDisplayYMinimum=-0.60000000000000009  ActiveDisplayYMaximum=0.60000000000000009  DataLoggingVariableName=ScopeData6  DataLoggingSaveFormat=Array
  Scope3 : Scope  Commented=on  NumInputPorts=2
      settings: TimeSpan=14.81551052143918  ActiveDisplayYMinimum=-4  ActiveDisplayYMaximum=3  DataLoggingVariableName=ScopeData7  DataLoggingSaveFormat=Array
  Sum1 : Sum  Inputs=|+++
  Sum4 : Sum  Inputs=|++
  Sum5 : Sum  Inputs=|++
  To Workspace : ToWorkspace  VariableName=yinc_lqr  SaveFormat=Timeseries  SampleTime=-1
  To Workspace3 : ToWorkspace  VariableName=yinc_hat  SaveFormat=Timeseries  SampleTime=-1
  n(1) : dspsrcs4/Random Source  SrcType=Gaussian  NormMethod=Ziggurat  CltLength=12  MinVal=0  MaxVal=1  MeanVal=0  VarVal=0.1  RepMode=Not repeatable  rawSeed=1  IsInherit=off  SampMode=Continuous  SampTime=1  SampFrame=1  DataType=Double  OutComplex=Real  OutputFrames=on
  n(1)3 : dspsrcs4/Random Source  SrcType=Gaussian  NormMethod=Ziggurat  CltLength=12  MinVal=0  MaxVal=1  MeanVal=0  VarVal=0.1  RepMode=Not repeatable  rawSeed=1  IsInherit=off  SampMode=Continuous  SampTime=1  SampFrame=1  DataType=Double  OutComplex=Real  OutputFrames=on
  n(2) : dspsrcs4/Random Source  SrcType=Gaussian  NormMethod=Ziggurat  CltLength=12  MinVal=0  MaxVal=1  MeanVal=0  VarVal=0.1  RepMode=Not repeatable  rawSeed=1  IsInherit=off  SampMode=Continuous  SampTime=1  SampFrame=1  DataType=Double  OutComplex=Real  OutputFrames=on
  yinc_hat : Outport
  wires:
  B/1 -> Sum1/2
  A/1 -> Sum1/1
  Sum1/1 -> Integrator/1
  Integrator/1 -> C/1, A/1
  n(1)/1 -> Mux/1
  n(2)/1 -> Mux/2
  Mux/1 -> E/1
  Kalman Filter/1 -> To Workspace3/1, yinc_hat/1, K_lqr/1, Scope2/1
  Kalman Filter/2 -> Scope3/1
  E/1 -> Sum1/3
  n(1)3/1 -> Sum4/1
  C/1 -> Sum4/2
  Sum4/1 -> Scope3/2, Kalman Filter/2, To Workspace/1
  Sum5/1 -> Kalman Filter/1, B/1
  K_lqr/1 -> Sum5/2
  incipient fault/1 -> Sum5/1

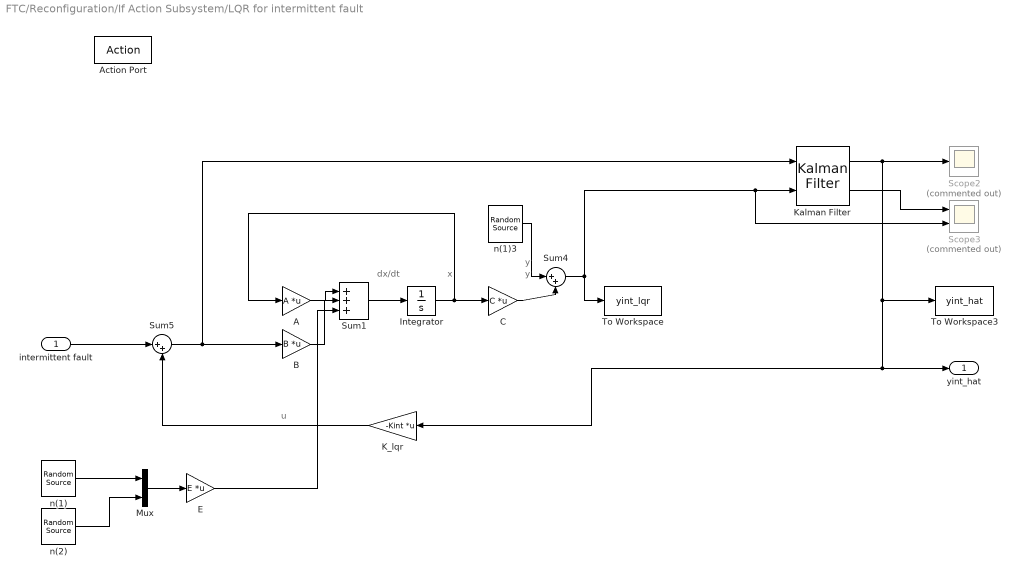
== system FTC/Reconfiguration/If Action Subsystem/LQR for intermittent fault ==
  note: u
  note: y
  note: x
  note: dx/dt
  note: y
  intermittent fault : Inport
  Action Port : ActionPort  ActionPortLabel=elseif { }
  A : Gain  Gain=A  Multiplication=Matrix(K*u)
  B : Gain  Gain=B  Multiplication=Matrix(K*u)
  C : Gain  Gain=C  Multiplication=Matrix(K*u)
  E : Gain  Gain=E  Multiplication=Matrix(K*u)
  Integrator : Integrator  InitialCondition=[2;0;0;0;0]
  K_lqr : Gain  Gain=-Kint  Multiplication=Matrix(K*u)
  Kalman Filter : ctrlSharedLib/Kalman Filter  TimeDomain=Continuous-Time  UseCurrentEstimator=on  ModelSource=Individual A, B, C, D matrices  ModelSourceVariable=ss(0.95,1,1,0,1)  A=A  B=B  C=C  D=zeros(5,2)  NumberOfStates=1  NumberOfInputs=1  NumberOfOutputs=1  InitialEstimateSource=Dialog  X0=zeros(5,1)  P0=10  UseK=off  UseGH=off  NumberOfProcessNoiseInputs=1  G=1  TimeInvariantG=on  H=0  TimeInvariantH=on  Q=0.001*eye(5)  TimeInvariantQ=on  R=0.001*eye(5)  TimeInvariantR=on  N=0  TimeInvariantN=on  AddInputPort=on  AddEnablePort=off  ExternalReset=none  OutputEstimatedY=on  OutputP=off  Ts=-1
  Mux : Mux  Inputs=2
  Scope2 : Scope  Commented=on
      settings: TimeSpan=14.81551052143918  ActiveDisplayYMinimum=-0.60000000000000009  ActiveDisplayYMaximum=0.60000000000000009  DataLoggingVariableName=ScopeData8  DataLoggingSaveFormat=Array
  Scope3 : Scope  Commented=on  NumInputPorts=2
      settings: TimeSpan=14.81551052143918  ActiveDisplayYMinimum=-4  ActiveDisplayYMaximum=3  DataLoggingVariableName=ScopeData14  DataLoggingSaveFormat=Array
  Sum1 : Sum  Inputs=|+++
  Sum4 : Sum  Inputs=|++
  Sum5 : Sum  Inputs=|++
  To Workspace : ToWorkspace  VariableName=yint_lqr  SaveFormat=Timeseries  SampleTime=-1
  To Workspace3 : ToWorkspace  VariableName=yint_hat  SaveFormat=Timeseries  SampleTime=-1
  n(1) : dspsrcs4/Random Source  SrcType=Gaussian  NormMethod=Ziggurat  CltLength=12  MinVal=0  MaxVal=1  MeanVal=0  VarVal=0.1  RepMode=Not repeatable  rawSeed=1  IsInherit=off  SampMode=Continuous  SampTime=1  SampFrame=1  DataType=Double  OutComplex=Real  OutputFrames=on
  n(1)3 : dspsrcs4/Random Source  SrcType=Gaussian  NormMethod=Ziggurat  CltLength=12  MinVal=0  MaxVal=1  MeanVal=0  VarVal=0.1  RepMode=Not repeatable  rawSeed=1  IsInherit=off  SampMode=Continuous  SampTime=1  SampFrame=1  DataType=Double  OutComplex=Real  OutputFrames=on
  n(2) : dspsrcs4/Random Source  SrcType=Gaussian  NormMethod=Ziggurat  CltLength=12  MinVal=0  MaxVal=1  MeanVal=0  VarVal=0.1  RepMode=Not repeatable  rawSeed=1  IsInherit=off  SampMode=Continuous  SampTime=1  SampFrame=1  DataType=Double  OutComplex=Real  OutputFrames=on
  yint_hat : Outport
  wires:
  B/1 -> Sum1/2
  A/1 -> Sum1/1
  Sum1/1 -> Integrator/1
  Integrator/1 -> C/1, A/1
  n(1)/1 -> Mux/1
  n(2)/1 -> Mux/2
  Mux/1 -> E/1
  Kalman Filter/1 -> Scope2/1, To Workspace3/1, yint_hat/1, K_lqr/1
  Kalman Filter/2 -> Scope3/1
  E/1 -> Sum1/3
  n(1)3/1 -> Sum4/1
  C/1 -> Sum4/2
  Sum4/1 -> Scope3/2, Kalman Filter/2, To Workspace/1
  Sum5/1 -> Kalman Filter/1, B/1
  K_lqr/1 -> Sum5/2
  intermittent fault/1 -> Sum5/1

== matlab function FTC/Fault Detection/MATLAB Function ==
  data: r_fault input; d1 output; d2 output; d3 output; d4 output; r_no_fault input
function [d1,d2,d3,d4]  = fcn(r_fault,r_no_fault)
%#codegen
% S=zeros(4,1000);
S=0;
d1=0;
d2=0;
d3=0;
d4=0;


temp=0;
temp2=0;

n=length(r_fault);

sigma1=var(r_no_fault);
% M=0.05;
M=0.0120;
temp=S;
temp2=r_fault-M/2;
alpha=0.2;%the false alarm probability
beta=0.2;%the missed alarm probability
a=log((1-beta)/alpha);%upper threshold limit
b=log(beta/(1-alpha));%lower threshold limit

% if (r_fault(1)>up || r_fault(1)<low)
%     d1=1;
%     %     disp(' Fault in state 1 at time:')
%
%
%
% else
%     d1=0;
%     %     disp('No Fault in state 1 at time:')
%
% end
% if (r_fault(2)>up || r_fault(2)<low)
%     d2=1;
%     %     disp(' Fault in state 2 at time:')
%
% else
%     d2=0;
%     %     disp(' No Fault in state 2 at time:')
%
%
% end
% if (r_fault(3)>up || r_fault(3)<low)
%     d3=1;
%     %     disp(' Fault in state 3 at time:')
%
% else
%     d3=0;
%     %     disp(' No Fault in state 3 at time:')
%
%
% end
%
% if (r_fault(4)>up || r_fault(4)<low)
%     d4=1;
%     %     disp(' Fault in state 4 at time:')
%
% else
%     d4=0;
%     %     disp(' No Fault in state 4 at time:')
%
%
% end
% if (r_fault(5)>up || r_fault(5)<low)
%     d5=1;
%     disp(' Fault in state 5 at time:')
%
% else
%     d5=0;
%     disp(' No Fault in state 5 at time:')
%
%
% end


%%%%SPRT

S=(M./sigma1) *(temp2)+temp;%because residual has gaussian distribution
temp=S;

if S(1)<=b
    d1=0;%Accept H0
    
else
    if S(1)>=a
        d1=1;%Accept H1
        
    else
        d1=-1;
        
    end
end

if S(2)<=b
    d2=0;%Accept H0
    
else
    if S(2)>=a
        d2=1;%Accept H1
        
    else
        d2=-1;
        
    end
end

if S(3)<=b
    d3=0;%Accept H0
    
else
    if S(3)>=a
        d3=1;%Accept H1
        
    else
        d3=-1;
        
    end
end

if S(4)<=b
    d4=0;%Accept H0
    
else
    if S(4)>=a
        d4=1;%Accept H1
        
    else
        d4=-1;
        
    end
end


end
